simulink model "ex1"  (R2021b)
settings: Solver=VariableStepAuto  StartTime=0.0  StopTime=10.0  RelTol=1e-3
values from neighbouring files (symbols this model uses):
  den_Grz = conv(dz, [1 -1])    [Rezolvare.m]
  num_Grz = conv(nz, [1 0])    [Rezolvare.m]
settings SolverCC: AlgebraicLoopSolver=TrustRegion
settings DebuggingCC: SFMachineParentedDataDiag=warning

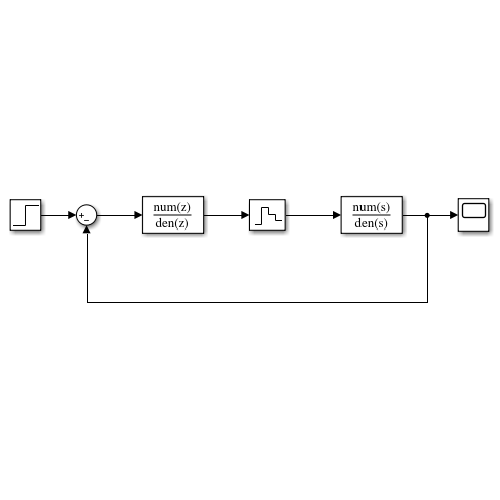
[thumbnail: Simulink's stored preview of the top-level diagram]
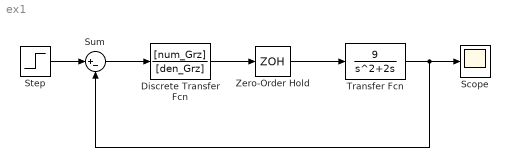
== system ex1 ==
  Discrete Transfer Fcn : DiscreteTransferFcn  Numerator=[num_Grz]  Denominator=[den_Grz]
  Scope : Scope
  Step : Step  SampleTime=0.1
  Sum : Sum  Inputs=|+-  SampleTime=0.1
  Transfer Fcn : TransferFcn  Numerator=[9]  Denominator=[1 2 0]
  Zero-Order Hold : ZeroOrderHold  SampleTime=-1
  wires:
  Step/1 -> Sum/1
  Sum/1 -> Discrete Transfer Fcn/1
  Discrete Transfer Fcn/1 -> Zero-Order Hold/1
  Zero-Order Hold/1 -> Transfer Fcn/1
  Transfer Fcn/1 -> Sum/2, Scope/1
